simulink model "ssc_fuel_cell_02"  (R2021b)
settings: Solver=VariableStepAuto  StartTime=0.0  StopTime=2000  RelTol=1e-3  AbsTol=1e-3
model workspace: external: MATLAB File ssc_fuel_cell_parameters.m (data not in the file)
undefined symbols (not defined in the file or in its folder): anode_tube_D, cathode_tube_D, comp_rpm_TLU, coolant_num_layers, coolant_num_passes, coolant_tube_D, coolant_w_channels, drive_cycle_power, drive_cycle_time, env_p, env_T, N2_T, radiator_air_area_fins, radiator_air_area_primary, radiator_eta_fin, radiator_N_tubes, radiator_rho, radiator_t_wall, radiator_tube_H, radiator_W, stack_alpha, stack_area, stack_iL, stack_io, stack_mea_rho, stack_num_cells, stack_num_channels, stack_t_gdl, stack_t_membrane, stack_w_channels
libraries: fl_lib x88, nesl_utility x23, slpidlib x2, simulink x1
(part 3 of 3)

== system ssc_fuel_cell_02/Cooling System/Coolant Tank ==
  Coolant Volume : fl_lib/Thermal Liquid/Elements/Translational Mechanical Converter (TL)  mech_orientation=foundation.enum.MechOrientationTranslational.Positive  displacement_spec=foundation.enum.DisplacementSpec.Calculate  x0=x_init m  interface_area=A m^2  dead_volume=A * 0.001 m^3  environment_spec=foundation.enum.pressure_spec.atmospheric  environment_pressure=0.101325 MPa  dynamic_compressibility=simscape.enum.onoff.off  p0=env_p MPa  T0=env_T degC
      settings: SourceProductBaseCode=SS  InternalSimscapePortConfiguration="{\"Bottom\":[],\"Left\":[{\"id\":\"A\",\"label\":\"A\",\"type\":\"foundation.thermal_liquid.thermal_liquid\"},{\"id\":\"C\",\"label\":\"C\",\"type\":\"foundation.mechanical.translational.translational\"},{\"id\":\"H\",\"label\":\"H\",\"type\":\"foundation.thermal.thermal\"}],\"Right\":[{\"id\":\"R\",\"label\":\"R\",\"type\":\"foundation.mechanical.translational.translational\"}],\"Top\":[]}"
  Mechanical Translational Reference : fl_lib/Mechanical/Translational Elements/Mechanical Translational Reference
  Perfect Insulator : fl_lib/Thermal/Thermal Elements/Perfect Insulator  T_specify=off  T_priority=None  T=0 K  T_nominal_specify=off  T_nominal_unit=K  T_nominal_value=1
  Translational Free End : fl_lib/Mechanical/Translational Elements/Translational Free End  v_specify=off  v_priority=None  v=0 m/s  v_nominal_specify=off  v_nominal_unit=m/s  v_nominal_value=1
      settings: SourceProductBaseCode=SS  InternalSimscapePortConfiguration="{\"Bottom\":[],\"Left\":[{\"id\":\"V\",\"label\":\"\",\"type\":\"foundation.mechanical.translational.translational\"}],\"Right\":[],\"Top\":[]}"
  T : PMIOPort  Side=Right
  connections:
  Coolant Volume/LConn1 -- T/RConn1
  Mechanical Translational Reference/LConn1 -- Coolant Volume/LConn2
  Translational Free End/LConn1 -- Coolant Volume/RConn1
  Perfect Insulator/LConn1 -- Coolant Volume/LConn3

== system ssc_fuel_cell_02/Cooling System/Pump Control ==
  T_set : Inport
  T_meas : Inport  Port=2
  Control Signals : Scope  NumInputPorts=2
  Mux : Mux  Inputs=2
  Mux1 : Mux  Inputs=2
  PID Controller : slpidlib/PID Controller  Controller=PI  Form=Ideal  TimeDomain=Continuous-time  UseExternalTs=off  SampleTime=-1  IntegratorMethod=Forward Euler  FilterMethod=Forward Euler  ControllerParametersSource=internal  P=0.1  I=0.01  D=0  UseFilter=on  N=100  TunerSelectOption=Transfer Function Based (PID Tuner App)  InitialConditionSource=internal  InitialConditionForIntegrator=0  InitialConditionForFilter=0  DifferentiatorICPrevScaledInput=0  ExternalReset=none  TrackingMode=off  Kt=1  LimitOutput=on  SatLimitsSource=internal  UpperSaturationLimit=1  LowerSaturationLimit=0  LinearizeAsGain=on  AntiWindupMode=back-calculation  Kb=0.1  POutMin=[]  POutMax=[]  IOutMin=[]  IOutMax=[]  DOutMin=[]  DOutMax=[]  NOutMin=[]  NOutMax=[]  SumOutMin=[]  SumOutMax=[]  SaturationOutMin=[]  SaturationOutMax=[]  PParamMin=[]  PParamMax=[]  IParamMin=[]  IParamMax=[]  DParamMin=[]  DParamMax=[]  NParamMin=[]  NParamMax=[]  KbParamMin=[]  KbParamMax=[]  KtParamMin=[]  KtParamMax=[]  KbOutMin=[]  KbOutMax=[]  KtOutMin=[]  KtOutMax=[]  IntegratorOutMin=[]  IntegratorOutMax=[]  FilterOutMin=[]  FilterOutMax=[]  SumI1OutMin=[]  SumI1OutMax=[]  SumI2OutMin=[]  SumI2OutMax=[]  SumI3OutMin=[]  SumI3OutMax=[]  SumI4OutMin=[]  SumI4OutMax=[]  SumDOutMin=[]  SumDOutMax=[]  DifferentiatorOutMin=[]  DifferentiatorOutMax=[]  FilterDiffOutCoefMin=[]  FilterDiffOutCoefMax=[]  ReciprocalOutMin=[]  ReciprocalOutMax=[]  SumDenOutMin=[]  SumDenOutMax=[]  SumNumOutMin=[]  SumNumOutMax=[]  DivideOutMin=[]  DivideOutMax=[]  UdiffTsProdOutMin=[]  UdiffTsProdOutMax=[]  NTsProdOutMin=[]  NTsProdOutMax=[]  UintegralTsProdOutMin=[]  UintegralTsProdOutMax=[]  UngainTsProdOutMin=[]  UngainTsProdOutMax=[]  IntegratorContinuousStateAttributes=''  IntegratorStateMustResolveToSignalObject=off  IntegratorRTWStateStorageClass=Auto  FilterContinuousStateAttributes=''  FilterStateMustResolveToSignalObject=off  FilterRTWStateStorageClass=Auto  ParallelPVariant=Passthrough  IdealPVariant=InternalParameters  IVariant=InternalParameters  DVariant=Disabled  IntegratorVariant=Continuous  SatVariant=Enabled  AWVariant=BackCalculation  PCopyVariant=Disabled  TRVariant=Disabled  FdbkBlocksVariant=Forward  IdealPFdbkVariant=Disabled  SatFdbkVariant=Disabled  DerivativeFilterVariant=Disabled  NVariant=Disabled  NCopyVariant=Disabled_SignalSpec  FilterICVariant=Disabled  IntegratorICVariant=InternalICs  ExternalResetVariant=Disabled  TRSumVariant=Passthrough  SumFdbkVariant=Disabled  SumVariant=Sum_PI  TsampFilterVariant=InternalTs  TsampNgainVariant=Passthrough  TsampIntegralVariant=Passthrough  ExternalSaturationOutDataTypeStr=Inherit: Same as second input
  Sum : Sum  Inputs=|-+
  Transfer Fcn : TransferFcn  Denominator=[2 1]
  cmd : Outport
  wires:
  Transfer Fcn/1 -> Mux1/2, cmd/1
  T_set/1 -> Mux/1, Sum/1
  T_meas/1 -> Mux/2, Sum/2
  Sum/1 -> PID Controller/1
  PID Controller/1 -> Mux1/1, Transfer Fcn/1
  Mux/1 -> Control Signals/1
  Mux1/1 -> Control Signals/2

== system ssc_fuel_cell_02/Electrical Load/Inputs ==
  Drive Cycle Power Demand : Subsystem  VariantControl=Drive cycle
      settings: PortSchema="{\"entries\":[{\"content\":{\"sides\":[{\"content\":{\"connectorIds\":[\"LConn1\"]},\"type\":\"ConnectorPlacement.EquallySpacedRectSide\",\"uuid\":\"316ab41f-9548-4c29-941b-82cd3006a9cc\"},{\"content\":{\"connectorIds\":[],\"side\":\"RIGHT\"},\"type\":\"ConnectorPlacement.EquallySpacedRectSide\",\"uuid\":\"21ddf6a1-5f8a-47a4-ab15-3c27c3a556ce\"},{\"content\":{\"connectorIds\":[\"LConn2\"],\"side\":\"TOP\"},\"type\":\"ConnectorPlacement.EquallySpacedRectSide\",\"uuid\":\"59191a52-f145-4ac2-9cf2-0e0b54b3d2a8\"}]},\"type\":\"ConnectorPlacement.EquallySpacedConnector\",\"uuid\":\"e8f988fd-b412-4b1a-aaea-374cf82170cc\"}],\"packageUris\":[\"http://schema.mathworks.com/mf0/Connector/R2020b\"],\"version\":\"1.0\"}"
      mask Display:
      | plot(0, 0)
      | plot(100, 100)
      | 
      | mws = get_param(bdroot, 'ModelWorkspace');
      | x = getVariable(mws, 'drive_cycle_time');
      | y = getVariable(mws, 'drive_cycle_power');
      | 
      | plot(x/max(x)*80 + 10, y/max(y)*60 + 30)
  Ramp Current Demand : Subsystem  VariantControl=Ramp
      settings: PortSchema="{\"entries\":[{\"content\":{\"sides\":[{\"content\":{\"connectorIds\":[\"LConn1\"]},\"type\":\"ConnectorPlacement.EquallySpacedRectSide\",\"uuid\":\"316ab41f-9548-4c29-941b-82cd3006a9cc\"},{\"content\":{\"connectorIds\":[],\"side\":\"RIGHT\"},\"type\":\"ConnectorPlacement.EquallySpacedRectSide\",\"uuid\":\"21ddf6a1-5f8a-47a4-ab15-3c27c3a556ce\"},{\"content\":{\"connectorIds\":[\"LConn2\"],\"side\":\"TOP\"},\"type\":\"ConnectorPlacement.EquallySpacedRectSide\",\"uuid\":\"59191a52-f145-4ac2-9cf2-0e0b54b3d2a8\"}]},\"type\":\"ConnectorPlacement.EquallySpacedConnector\",\"uuid\":\"e8f988fd-b412-4b1a-aaea-374cf82170cc\"}],\"packageUris\":[\"http://schema.mathworks.com/mf0/Connector/R2020b\"],\"version\":\"1.0\"}"
      mask Display:
      | plot(0, 0)
      | plot(100, 100)
      | 
      | plot([20 40 80], [20 20 90])
  Step Current Demand : Subsystem  VariantControl=Step
      settings: PortSchema="{\"entries\":[{\"content\":{\"sides\":[{\"content\":{\"connectorIds\":[\"LConn1\"]},\"type\":\"ConnectorPlacement.EquallySpacedRectSide\",\"uuid\":\"316ab41f-9548-4c29-941b-82cd3006a9cc\"},{\"content\":{\"connectorIds\":[],\"side\":\"RIGHT\"},\"type\":\"ConnectorPlacement.EquallySpacedRectSide\",\"uuid\":\"21ddf6a1-5f8a-47a4-ab15-3c27c3a556ce\"},{\"content\":{\"connectorIds\":[\"LConn2\"],\"side\":\"TOP\"},\"type\":\"ConnectorPlacement.EquallySpacedRectSide\",\"uuid\":\"59191a52-f145-4ac2-9cf2-0e0b54b3d2a8\"}]},\"type\":\"ConnectorPlacement.EquallySpacedConnector\",\"uuid\":\"e8f988fd-b412-4b1a-aaea-374cf82170cc\"}],\"packageUris\":[\"http://schema.mathworks.com/mf0/Connector/R2020b\"],\"version\":\"1.0\"}"
      mask Display:
      | plot(0, 0)
      | plot(100, 100)
      | 
      | plot([20 50 50 80], [20 20 80 80])
  i : PMIOPort  Side=Left
  v : PMIOPort  Port=2  Side=Left

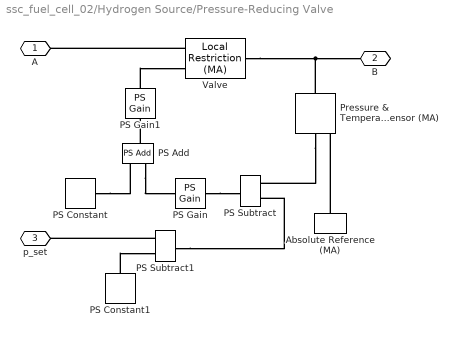
== system ssc_fuel_cell_02/Hydrogen Source/Pressure-Reducing Valve ==
  Absolute Reference (MA) : fl_lib/Moist Air/Elements/Absolute Reference (MA)
      settings: SourceProductBaseCode=SS
  PS Add : fl_lib/Physical Signals/Functions/PS Add
  PS Constant : fl_lib/Physical Signals/Sources/PS Constant  constant=r_max^2
  PS Constant1 : fl_lib/Physical Signals/Sources/PS Constant  constant=p_range MPa
  PS Gain : fl_lib/Physical Signals/Functions/PS Gain  gain=(r_min^2 - r_max^2)/p_range 1/MPa
  PS Gain1 : fl_lib/Physical Signals/Functions/PS Gain  gain=pi*D^2/4 m^2
  PS Subtract : fl_lib/Physical Signals/Functions/PS Subtract
  PS Subtract1 : fl_lib/Physical Signals/Functions/PS Subtract
  Pressure & Temperature Sensor (MA) : fl_lib/Moist Air/Sensors/Pressure & Temperature Sensor (MA)
      settings: SourceProductBaseCode=SS  InternalSimscapePortConfiguration="{\"Bottom\":[],\"Left\":[{\"id\":\"A\",\"label\":\"A\",\"type\":\"foundation.moist_air.moist_air\"}],\"Right\":[{\"id\":\"B\",\"label\":\"B\",\"type\":\"foundation.moist_air.moist_air\"},{\"id\":\"P\",\"label\":\"P\",\"type\":\"output\"},{\"id\":\"T\",\"label\":\"T\",\"type\":\"output\"}],\"Top\":[]}"
  Valve : fl_lib/Moist Air/Elements/Local Restriction (MA)  restriction_type=foundation.enum.restriction_type.variable  restriction_area=0.001 m^2  min_area=pi*(r_min*D)^2/4 m^2  max_area=pi*(r_max*D)^2/4 m^2  area=pi*D^2/4 m^2  Cd=0.64  B_lam=0.999
      settings: SourceProductBaseCode=SS
  A : PMIOPort  Side=Left
  B : PMIOPort  Port=2  Side=Right
  p_set : PMIOPort  Port=3  Side=Left
  connections:
  PS Constant1/RConn1 -- PS Subtract1/LConn2
  PS Subtract1/LConn1 -- p_set/RConn1
  PS Subtract1/RConn1 -- PS Subtract/LConn2
  PS Constant/RConn1 -- PS Add/LConn1
  PS Add/LConn2 -- PS Gain/RConn1
  PS Add/RConn1 -- PS Gain1/LConn1
  PS Gain/LConn1 -- PS Subtract/RConn1
  Pressure & Temperature Sensor (MA)/RConn2 -- PS Subtract/LConn1
  PS Gain1/RConn1 -- Valve/LConn2
  Absolute Reference (MA)/LConn1 -- Pressure & Temperature Sensor (MA)/RConn1
  Pressure & Temperature Sensor (MA)/LConn1 -- B/RConn1 -- Valve/RConn1
  Valve/LConn1 -- A/RConn1

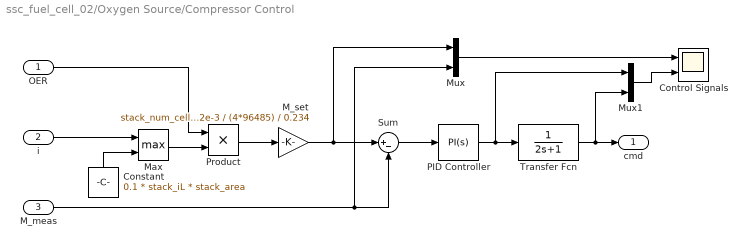
== system ssc_fuel_cell_02/Oxygen Source/Compressor Control ==
  OER : Inport
  i : Inport  Port=2
  M_meas : Inport  Port=3
  Constant : Constant  Value=0.1 * stack_iL * stack_area
  Control Signals : Scope  NumInputPorts=2
  M_set : Gain  Gain=stack_num_cells * 32e-3 / (4*96485) / 0.234
  Max : MinMax  Function=max  Inputs=2  ZeroCross=off
  Mux : Mux  Inputs=2
  Mux1 : Mux  Inputs=2
  PID Controller : slpidlib/PID Controller  Controller=PI  Form=Ideal  TimeDomain=Continuous-time  UseExternalTs=off  SampleTime=-1  IntegratorMethod=Forward Euler  FilterMethod=Forward Euler  ControllerParametersSource=internal  P=5  I=0.5  D=0  UseFilter=on  N=100  TunerSelectOption=Transfer Function Based (PID Tuner App)  InitialConditionSource=internal  InitialConditionForIntegrator=0  InitialConditionForFilter=0  DifferentiatorICPrevScaledInput=0  ExternalReset=none  TrackingMode=off  Kt=1  LimitOutput=on  SatLimitsSource=internal  UpperSaturationLimit=1  LowerSaturationLimit=0  LinearizeAsGain=on  AntiWindupMode=back-calculation  Kb=1  POutMin=[]  POutMax=[]  IOutMin=[]  IOutMax=[]  DOutMin=[]  DOutMax=[]  NOutMin=[]  NOutMax=[]  SumOutMin=[]  SumOutMax=[]  SaturationOutMin=[]  SaturationOutMax=[]  PParamMin=[]  PParamMax=[]  IParamMin=[]  IParamMax=[]  DParamMin=[]  DParamMax=[]  NParamMin=[]  NParamMax=[]  KbParamMin=[]  KbParamMax=[]  KtParamMin=[]  KtParamMax=[]  KbOutMin=[]  KbOutMax=[]  KtOutMin=[]  KtOutMax=[]  IntegratorOutMin=[]  IntegratorOutMax=[]  FilterOutMin=[]  FilterOutMax=[]  SumI1OutMin=[]  SumI1OutMax=[]  SumI2OutMin=[]  SumI2OutMax=[]  SumI3OutMin=[]  SumI3OutMax=[]  SumI4OutMin=[]  SumI4OutMax=[]  SumDOutMin=[]  SumDOutMax=[]  DifferentiatorOutMin=[]  DifferentiatorOutMax=[]  FilterDiffOutCoefMin=[]  FilterDiffOutCoefMax=[]  ReciprocalOutMin=[]  ReciprocalOutMax=[]  SumDenOutMin=[]  SumDenOutMax=[]  SumNumOutMin=[]  SumNumOutMax=[]  DivideOutMin=[]  DivideOutMax=[]  UdiffTsProdOutMin=[]  UdiffTsProdOutMax=[]  NTsProdOutMin=[]  NTsProdOutMax=[]  UintegralTsProdOutMin=[]  UintegralTsProdOutMax=[]  UngainTsProdOutMin=[]  UngainTsProdOutMax=[]  IntegratorContinuousStateAttributes=''  IntegratorStateMustResolveToSignalObject=off  IntegratorRTWStateStorageClass=Auto  FilterContinuousStateAttributes=''  FilterStateMustResolveToSignalObject=off  FilterRTWStateStorageClass=Auto  ParallelPVariant=Passthrough  IdealPVariant=InternalParameters  IVariant=InternalParameters  DVariant=Disabled  IntegratorVariant=Continuous  SatVariant=Enabled  AWVariant=BackCalculation  PCopyVariant=Disabled  TRVariant=Disabled  FdbkBlocksVariant=Forward  IdealPFdbkVariant=Disabled  SatFdbkVariant=Disabled  DerivativeFilterVariant=Disabled  NVariant=Disabled  NCopyVariant=Disabled_SignalSpec  FilterICVariant=Disabled  IntegratorICVariant=InternalICs  ExternalResetVariant=Disabled  TRSumVariant=Passthrough  SumFdbkVariant=Disabled  SumVariant=Sum_PI  TsampFilterVariant=InternalTs  TsampNgainVariant=Passthrough  TsampIntegralVariant=Passthrough  ExternalSaturationOutDataTypeStr=Inherit: Same as second input
  Product : Product
  Sum : Sum  Inputs=|+-
  Transfer Fcn : TransferFcn  Denominator=[2 1]
  cmd : Outport
  wires:
  OER/1 -> Product/1
  Constant/1 -> Max/2
  i/1 -> Max/1
  Max/1 -> Product/2
  PID Controller/1 -> Mux1/1, Transfer Fcn/1
  Sum/1 -> PID Controller/1
  M_set/1 -> Sum/1, Mux/1
  Product/1 -> M_set/1
  M_meas/1 -> Mux/2, Sum/2
  Transfer Fcn/1 -> Mux1/2, cmd/1
  Mux/1 -> Control Signals/1
  Mux1/1 -> Control Signals/2

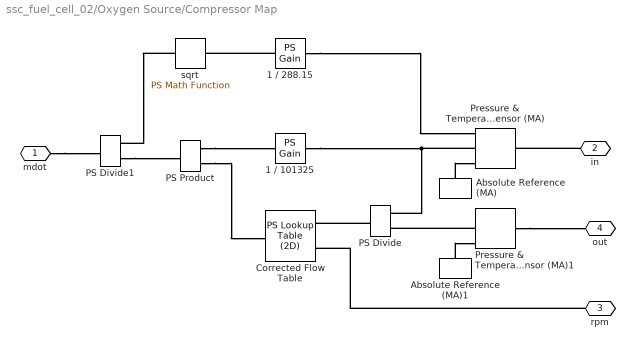
== system ssc_fuel_cell_02/Oxygen Source/Compressor Map ==
  1 / 101325 : fl_lib/Physical Signals/Functions/PS Gain  gain=1 / 101325 1/Pa
  1 / 288.15 : fl_lib/Physical Signals/Functions/PS Gain  gain=1 / 288.15 1/K
  Absolute Reference (MA) : fl_lib/Moist Air/Elements/Absolute Reference (MA)
      settings: SourceProductBaseCode=SS
  Absolute Reference (MA)1 : fl_lib/Moist Air/Elements/Absolute Reference (MA)
      settings: SourceProductBaseCode=SS
  Corrected Flow Table : fl_lib/Physical Signals/Lookup Tables/PS Lookup Table (2D)  x1=comp_p_ratio_TLU Pa/Pa  x2=comp_rpm_TLU rpm  f=comp_mdot_corr_TLU kg/s  interp_method=simscape.enum.interpolation.linear  extrap_method=simscape.enum.extrapolation.nearest
      settings: SourceProductBaseCode=SS
  PS Divide : fl_lib/Physical Signals/Functions/PS Divide
      settings: SourceProductBaseCode=SS
  PS Divide1 : fl_lib/Physical Signals/Functions/PS Divide
      settings: SourceProductBaseCode=SS
  PS Product : fl_lib/Physical Signals/Functions/PS Product
  Pressure & Temperature Sensor (MA) : fl_lib/Moist Air/Sensors/Pressure & Temperature Sensor (MA)
      settings: SourceProductBaseCode=SS  InternalSimscapePortConfiguration="{\"Bottom\":[],\"Left\":[{\"id\":\"A\",\"label\":\"A\",\"type\":\"foundation.moist_air.moist_air\"}],\"Right\":[{\"id\":\"B\",\"label\":\"B\",\"type\":\"foundation.moist_air.moist_air\"},{\"id\":\"P\",\"label\":\"P\",\"type\":\"output\"},{\"id\":\"T\",\"label\":\"T\",\"type\":\"output\"}],\"Top\":[]}"
  Pressure & Temperature Sensor (MA)1 : fl_lib/Moist Air/Sensors/Pressure & Temperature Sensor (MA)
      settings: SourceProductBaseCode=SS  InternalSimscapePortConfiguration="{\"Bottom\":[],\"Left\":[{\"id\":\"A\",\"label\":\"A\",\"type\":\"foundation.moist_air.moist_air\"}],\"Right\":[{\"id\":\"B\",\"label\":\"B\",\"type\":\"foundation.moist_air.moist_air\"},{\"id\":\"P\",\"label\":\"P\",\"type\":\"output\"},{\"id\":\"T\",\"label\":\"T\",\"type\":\"output\"}],\"Top\":[]}"
  sqrt : fl_lib/Physical Signals/Functions/PS Math Function  fcn_choice=foundation.enum.math_function.sqrt  v=1
      settings: SourceProductBaseCode=SS
  mdot : PMIOPort  Side=Left
  in : PMIOPort  Port=2  Side=Right
  rpm : PMIOPort  Port=3  Side=Right
  out : PMIOPort  Port=4  Side=Right
  connections:
  Pressure & Temperature Sensor (MA)1/LConn1 -- out/RConn1
  Absolute Reference (MA)/LConn1 -- Pressure & Temperature Sensor (MA)/RConn1
  in/RConn1 -- Pressure & Temperature Sensor (MA)/LConn1
  1 / 101325/LConn1 -- Pressure & Temperature Sensor (MA)/RConn2 -- PS Divide/LConn2
  rpm/RConn1 -- Corrected Flow Table/LConn2
  PS Divide/RConn1 -- Corrected Flow Table/LConn1
  1 / 288.15/LConn1 -- Pressure & Temperature Sensor (MA)/RConn3
  PS Product/LConn1 -- 1 / 101325/RConn1
  PS Product/LConn2 -- Corrected Flow Table/RConn1
  PS Divide1/LConn1 -- PS Product/RConn1
  1 / 288.15/RConn1 -- sqrt/LConn1
  sqrt/RConn1 -- PS Divide1/LConn2
  mdot/RConn1 -- PS Divide1/RConn1
  Absolute Reference (MA)1/LConn1 -- Pressure & Temperature Sensor (MA)1/RConn1
  Pressure & Temperature Sensor (MA)1/RConn2 -- PS Divide/LConn1

== system ssc_fuel_cell_02/Recirculation/Feedforward Control ==
  i : Inport
  Constant : Constant  Value=0.2
  Gain : Gain  Gain=0.8 / (stack_iL * stack_area)
  Saturation : Saturate  UpperLimit=1  LowerLimit=0
  Sum : Sum  Inputs=|++
  Transfer Fcn : TransferFcn  Denominator=[2 1]
  cmd : Outport
  wires:
  i/1 -> Gain/1
  Transfer Fcn/1 -> cmd/1
  Gain/1 -> Sum/1
  Constant/1 -> Sum/2
  Sum/1 -> Saturation/1
  Saturation/1 -> Transfer Fcn/1

== system ssc_fuel_cell_02/Electrical Load/Inputs/Drive Cycle Power Demand ==
  Clock : Clock
  PS Divide : fl_lib/Physical Signals/Functions/PS Divide
      settings: SourceProductBaseCode=SS
  PS-Simulink Converter : nesl_utility/PS-Simulink Converter  PhysicalDomain=network_engine_domain  SubClassName=ps_output  LeftPortType=input  RightPortType=output  PseudoPeriodic=off  Frequencies=[]  Unit=V  AffineConversion=off
      settings: SourceProductBaseCode=PW,SS
  PS-Simulink Converter1 : nesl_utility/PS-Simulink Converter  PhysicalDomain=network_engine_domain  SubClassName=ps_output  LeftPortType=input  RightPortType=output  PseudoPeriodic=off  Frequencies=[]  Unit=A  AffineConversion=off
      settings: SourceProductBaseCode=PW,SS
  Power (kW) : Lookup_n-D  NumberOfTableDimensions=1  BreakpointsForDimension1=drive_cycle_time  IndexSearchMethod=Linear search  BeginIndexSearchUsingPreviousIndexResult=on  Table=drive_cycle_power  ExtrapMethod=Clip  InternalRulePriority=Speed  RndMeth=Simplest  InputSameDT=on
  Simulink-PS Converter : nesl_utility/Simulink-PS Converter  PhysicalDomain=network_engine_domain  SubClassName=ps_input  LeftPortType=input  RightPortType=output  PseudoPeriodic=off  Frequencies=[]  NoiseDistribution=none  NoiseParameters=[]  Unit=kW  AffineConversion=off  FilteringAndDerivatives=provide  SimscapeFilterOrder=1  InputFilterTimeConstant=0.001  UdotUserProvided=0
      settings: SourceProductBaseCode=PW,SS
  i : PMIOPort  Side=Left
  v : PMIOPort  Port=2  Side=Left
  tag scope: i_stack=global, v_stack=global
  wires:
  Power (kW)/1 -> Simulink-PS Converter/1
  Clock/1 -> Power (kW)/1
  PS-Simulink Converter/1 -> [v_stack]
  PS-Simulink Converter1/1 -> [i_stack]
  connections:
  PS Divide/LConn1 -- Simulink-PS Converter/RConn1
  i/RConn1 -- PS Divide/RConn1 -- PS-Simulink Converter1/LConn1
  v/RConn1 -- PS-Simulink Converter/LConn1 -- PS Divide/LConn2

== system ssc_fuel_cell_02/Electrical Load/Inputs/Ramp Current Demand ==
  PS-Simulink Converter : nesl_utility/PS-Simulink Converter  PhysicalDomain=network_engine_domain  SubClassName=ps_output  LeftPortType=input  RightPortType=output  PseudoPeriodic=off  Frequencies=[]  Unit=V  AffineConversion=off
      settings: SourceProductBaseCode=PW,SS
  Ramp : simulink/Sources/Ramp  slope=-stack_iL * stack_area * (1 - 2e-6) / (2500 - 100)  start=1000  InitialOutput=stack_iL * stack_area * (1 - 2e-6) / (2500 - 100)*1000
  Simulink-PS Converter : nesl_utility/Simulink-PS Converter  PhysicalDomain=network_engine_domain  SubClassName=ps_input  LeftPortType=input  RightPortType=output  PseudoPeriodic=off  Frequencies=[]  NoiseDistribution=none  NoiseParameters=[]  Unit=A  AffineConversion=off  FilteringAndDerivatives=filter  SimscapeFilterOrder=1  InputFilterTimeConstant=0.001  UdotUserProvided=0
      settings: SourceProductBaseCode=PW,SS
  i : PMIOPort  Side=Left
  v : PMIOPort  Port=2  Side=Left
  tag scope: i_stack=global, v_stack=global
  wires:
  PS-Simulink Converter/1 -> [v_stack]
  Ramp/1 -> [i_stack], Simulink-PS Converter/1
  connections:
  Simulink-PS Converter/RConn1 -- i/RConn1
  v/RConn1 -- PS-Simulink Converter/LConn1

== system ssc_fuel_cell_02/Electrical Load/Inputs/Step Current Demand ==
  PS-Simulink Converter : nesl_utility/PS-Simulink Converter  PhysicalDomain=network_engine_domain  SubClassName=ps_output  LeftPortType=input  RightPortType=output  PseudoPeriodic=off  Frequencies=[]  Unit=V  AffineConversion=off
      settings: SourceProductBaseCode=PW,SS
  Simulink-PS Converter : nesl_utility/Simulink-PS Converter  PhysicalDomain=network_engine_domain  SubClassName=ps_input  LeftPortType=input  RightPortType=output  PseudoPeriodic=off  Frequencies=[]  NoiseDistribution=none  NoiseParameters=[]  Unit=A  AffineConversion=off  FilteringAndDerivatives=provide  SimscapeFilterOrder=1  InputFilterTimeConstant=0.001  UdotUserProvided=0
      settings: SourceProductBaseCode=PW,SS
  Step : Step  Time=500  Before=1e-6 * stack_iL * stack_area  After=0.5 * stack_iL * stack_area  SampleTime=0
  i : PMIOPort  Side=Left
  v : PMIOPort  Port=2  Side=Left
  tag scope: i_stack=global, v_stack=global
  wires:
  Step/1 -> [i_stack], Simulink-PS Converter/1
  PS-Simulink Converter/1 -> [v_stack]
  connections:
  Simulink-PS Converter/RConn1 -- i/RConn1
  PS-Simulink Converter/LConn1 -- v/RConn1
